simulink model "B1sistemaNonLineareRegolato"  (R2022b)
settings: Solver=ode45  StartTime=0.0  StopTime=100  RelTol=1e-3
values from neighbouring files (symbols this model uses):
  alfa = 0.2    [ProgettoCATFinale.m]
  beta = 0.3    [ProgettoCATFinale.m]
  gamma = 0.3    [ProgettoCATFinale.m]
  K = 200    [ProgettoCATFinale.m]
  m_r = 0.15    [ProgettoCATFinale.m]
  m_s = 0.7    [ProgettoCATFinale.m]
  r_r = 1.3    [ProgettoCATFinale.m]
  r_s = 1.5    [ProgettoCATFinale.m]
  RR = RR_s*RR_lf*RR_hf    [ProgettoCATFinale.m]
  sample_time = 0.0001    [ProgettoCATFinale.m]
  u_e = 0    [ProgettoCATFinale.m]
  WW = -2    [ProgettoCATFinale.m]
  x0 = [95; 102]    [ProgettoCATFinale.m]
  xe2 = n_r_e    (= 100)    [ProgettoCATFinale.m]
libraries: simulink x2
settings Model: Creator=nanni  LastModifiedBy=nanni

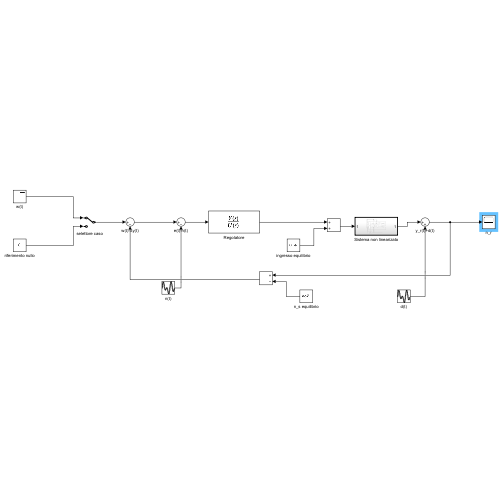
[thumbnail: Simulink's stored preview of the top-level diagram]
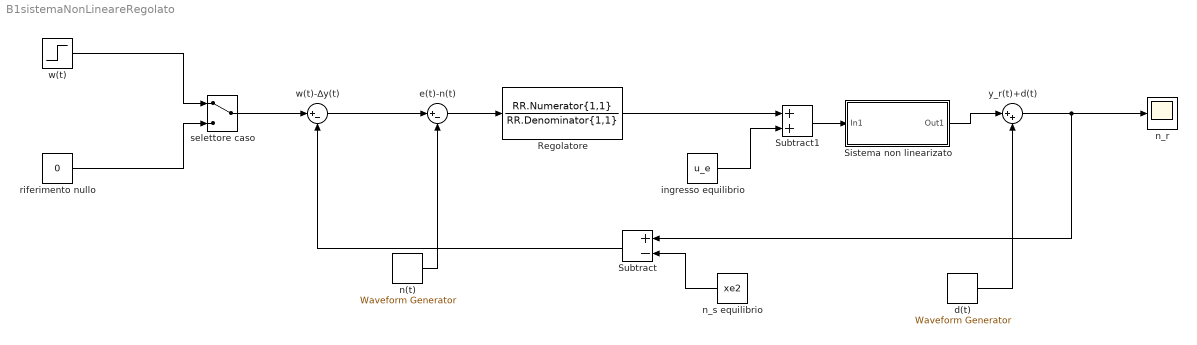
== system B1sistemaNonLineareRegolato ==
  Regolatore : TransferFcn  Numerator=RR.Numerator{1,1}  Denominator=RR.Denominator{1,1}  ParameterTunability=Unconstrained  ContinuousStateAttributes='regolatore'
  Sistema non linearizato : Subsystem  TreatAsAtomicUnit=on
  Subtract : Sum  Inputs=+-
  Subtract1 : Sum
  d(t) : simulink/Sources/Waveform Generator  OutMin=[]  OutMax=[]  OutDataTypeStr=double  SelectedSignal=1  Signals=sin(0.3,0.0125,0)+sin(0.3,0.0250,0)+sin(0.3,0.0375,0)+sin(0.3,0.05,0)  BlockNames=MultiportSwitch_9055b06cbe24481  SampleTime=sample_time
  e(t)-n(t) : Sum  Inputs=|+-
  ingresso equilibrio : Constant  Value=u_e
  n(t) : simulink/Sources/Waveform Generator  OutMin=[]  OutMax=[]  OutDataTypeStr=double  SelectedSignal=1  Signals=sin(0.2,10000,0)+sin(0.2,20000,0)+sin(0.2,30000,0)+sin(0.2,40000,0)  BlockNames=MultiportSwitch_697720dccfeb45c  SampleTime=sample_time
  n_r : Scope
  n_s equilibrio : Constant  Value=xe2
  riferimento nullo : Constant  Value=0
  selettore caso : ManualSwitch
  w(t) : Step  Time=0.001  After=WW  SampleTime=sample_time
  w(t)-∆y(t) : Sum  Inputs=|+-
  y_r(t)+d(t) : Sum  Inputs=|++
  wires:
  n(t)/1 -> e(t)-n(t)/2
  w(t)-∆y(t)/1 -> e(t)-n(t)/1
  e(t)-n(t)/1 -> Regolatore/1
  Sistema non linearizato/1(Out1) -> y_r(t)+d(t)/1
  d(t)/1 -> y_r(t)+d(t)/2
  y_r(t)+d(t)/1 -> Subtract/1, n_r/1
  n_s equilibrio/1 -> Subtract/2
  Subtract/1 -> w(t)-∆y(t)/2
  Subtract1/1 -> Sistema non linearizato/1(In1)
  ingresso equilibrio/1 -> Subtract1/2
  Regolatore/1 -> Subtract1/1
  selettore caso/1 -> w(t)-∆y(t)/1
  w(t)/1 -> selettore caso/1
  riferimento nullo/1 -> selettore caso/2

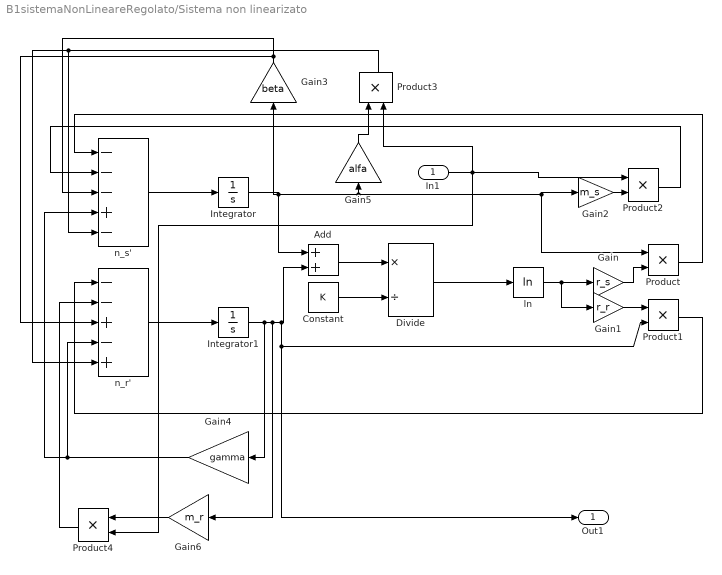
== system B1sistemaNonLineareRegolato/Sistema non linearizato ==
  In1 : Inport
  Add : Sum
  Constant : Constant  Value=K
  Divide : Product  Inputs=*/
  Gain : Gain  Gain=r_s
  Gain1 : Gain  Gain=r_r
  Gain2 : Gain  Gain=m_s
  Gain3 : Gain  Gain=beta
  Gain4 : Gain  Gain=gamma
  Gain5 : Gain  Gain=alfa
  Gain6 : Gain  Gain=m_r
  Integrator : Integrator  InitialCondition=x0(1,1)
  Integrator1 : Integrator  InitialCondition=x0(2,1)
  Product{,1..4} (5 alike) : Product
  ln : Math  Operator=log
  n_r' : Sum  Inputs=--+-+
  n_s' : Sum  Inputs=---+-
  Out1 : Outport
  wires:
  n_s'/1 -> Integrator/1
  n_r'/1 -> Integrator1/1
  Integrator/1 -> Gain3/1, Gain5/1, Gain2/1, Product/1, Add/1
  Integrator1/1 -> Gain4/1, Gain6/1, Product1/2, Out1/1, Add/2
  Add/1 -> Divide/1
  Constant/1 -> Divide/2
  Divide/1 -> ln/1
  ln/1 -> Gain1/1, Gain/1
  Gain/1 -> Product/2
  Product/1 -> n_s'/1
  Gain1/1 -> Product1/1
  Product1/1 -> n_r'/1
  In1/1 -> Product4/2, Product2/1, Product3/2
  Gain2/1 -> Product2/2
  Product2/1 -> n_s'/2
  Gain3/1 -> n_s'/3, n_r'/3
  Gain4/1 -> n_s'/4, n_r'/4
  Gain5/1 -> Product3/1
  Gain6/1 -> Product4/1
  Product4/1 -> n_r'/2
  Product3/1 -> n_r'/5, n_s'/5
